simulink model "generateDisturbance"  (R2019a)
settings: Solver=VariableStepAuto  StartTime=0.0  StopTime=2*tsim  MaxStep=1e-4  RelTol=1e-12  EnableMultiTasking=on
values from neighbouring files (symbols this model uses):
  h = 0.01    [aa_MAGLEV_changeSlope.m]
settings Model: Creator=alcasfra  LastModifiedBy=alcas
settings SolverCC: AlgebraicLoopSolver=LineSearch
settings DataIOCC: ReturnWorkspaceOutputs=off
settings OptimizationCC: LifeSpan=inf
settings DebuggingCC: SFUnexpectedBacktrackingDiag=warning  SFNoUnconditionalDefaultTransitionDiag=warning  ArithmeticOperatorsInVariantConditions=warning
settings SFSimCC: SimUseLocalCustomCode=off
settings RTWCC: RTWUseLocalCustomCode=off
settings CodeAppCC: StateflowObjectComments=on
settings GRTTargetCC: TargetLangStandard=C89/C90 (ANSI)  GeneratePreprocessorConditionals=Disable all
settings ConfigComp: CovMetricSettings=dw  CovHtmlReporting=on  CovSaveCumulativeToWorkspaceVar=on  CovSaveSingleToWorkspaceVar=on  CovExternalEMLEnable=off

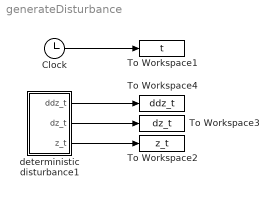
== system generateDisturbance ==
  Clock : Clock
  To Workspace1 : ToWorkspace  VariableName=t  SampleTime=h
      settings: Save2DSignal=2-D array (concatenate along first dimension)
  To Workspace2 : ToWorkspace  VariableName=z_t  SampleTime=h
      settings: Save2DSignal=2-D array (concatenate along first dimension)
  To Workspace3 : ToWorkspace  VariableName=dz_t  SampleTime=h
      settings: Save2DSignal=2-D array (concatenate along first dimension)
  To Workspace4 : ToWorkspace  VariableName=ddz_t  SampleTime=h
      settings: Save2DSignal=2-D array (concatenate along first dimension)
  deterministic disturbance1 : Subsystem
  wires:
  deterministic disturbance1/1(ddz_t) -> To Workspace4/1
  deterministic disturbance1/3(z_t) -> To Workspace2/1
  deterministic disturbance1/2(dz_t) -> To Workspace3/1
  Clock/1 -> To Workspace1/1

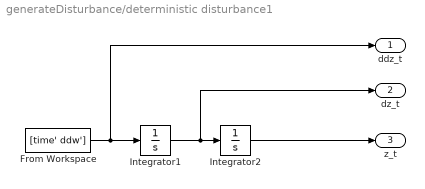
== system generateDisturbance/deterministic disturbance1 ==
  From Workspace : FromWorkspace  VariableName=[time' ddw']  SampleTime=0
  Integrator1 : Integrator
  Integrator2 : Integrator
  ddz_t : Outport
  dz_t : Outport  Port=2
  z_t : Outport  Port=3
  wires:
  Integrator2/1 -> z_t/1
  Integrator1/1 -> dz_t/1, Integrator2/1
  From Workspace/1 -> ddz_t/1, Integrator1/1
